simulink model "disk drive adaptive control"  (R2020a)
settings: Solver=VariableStepAuto  StartTime=0.0  StopTime=100  RelTol=1e-13  AbsTol=1e-8
InitFcn:
  | A1=2*rand(1);
  | A2=4*rand(1);
  | w1=1;w2=3;
  | phi1=2*pi*rand(1);
  | phi2=2*pi*rand(1);
  | Kp=1;
  | gamma=10;
  | A1ref=3;
  | A2ref=2;
  | w1ref=2;w2ref=sqrt(3);
  | phi1ref=0;
  | phi2ref=pi/4;
settings Model: Creator=Haris  LastModifiedBy=Haris

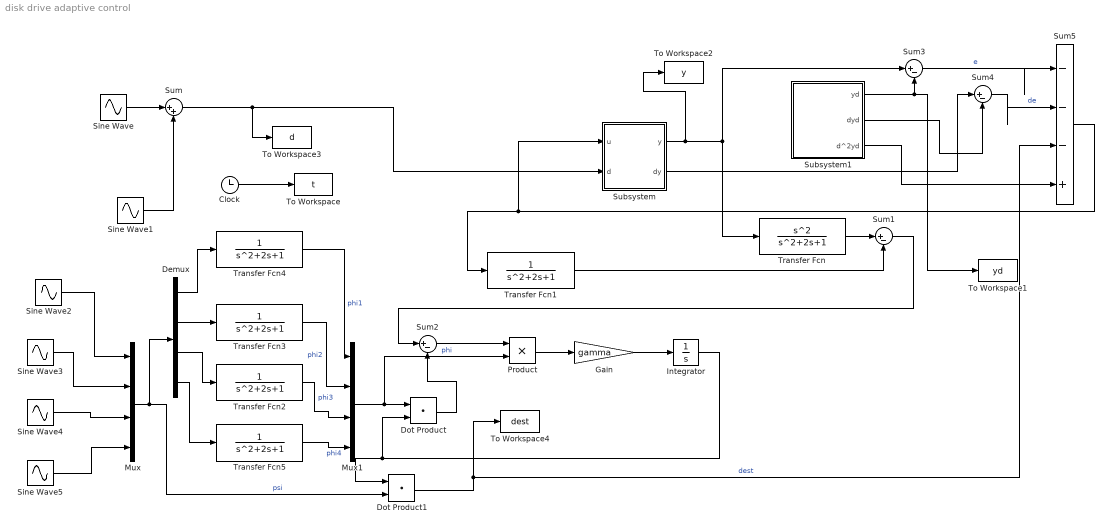
== system disk drive adaptive control ==
  Clock : Clock
  Demux : Demux
  Dot Product : DotProduct  InputSameDT=on  OutDataTypeStr=Inherit: Inherit via internal rule
  Dot Product1 : DotProduct  InputSameDT=on  OutDataTypeStr=Inherit: Inherit via internal rule
  Gain : Gain  Gain=gamma
  Integrator : Integrator  InitialCondition=[0;0;0;0]
  Mux : Mux
  Mux1 : Mux
  Product : Product
  Sine Wave : Sin  Amplitude=A1  Frequency=w1  Phase=phi1  SampleTime=0
  Sine Wave1 : Sin  Amplitude=A2  Frequency=w2  Phase=phi2  SampleTime=0
  Sine Wave2 : Sin  Frequency=w1  SampleTime=0
  Sine Wave3 : Sin  Frequency=w1  Phase=pi/2  SampleTime=0
  Sine Wave4 : Sin  Frequency=w2  SampleTime=0
  Sine Wave5 : Sin  Frequency=w2  Phase=pi/2  SampleTime=0
  Subsystem : Subsystem
  Subsystem1 : Subsystem
  Sum : Sum  Inputs=|++
  Sum{1..4} (4 alike) : Sum  Inputs=|+-
  Sum5 : Sum  Inputs=|---+
  To Workspace : ToWorkspace  VariableName=t  SampleTime=-1
  To Workspace1 : ToWorkspace  VariableName=yd  SampleTime=-1
  To Workspace2 : ToWorkspace  VariableName=y  SampleTime=-1
  To Workspace3 : ToWorkspace  VariableName=d  SampleTime=-1
  To Workspace4 : ToWorkspace  VariableName=dest  SampleTime=-1
  Transfer Fcn : TransferFcn  Numerator=[1 0 0]
  Transfer Fcn{1..5} (5 alike) : TransferFcn
  wires:
  Sine Wave/1 -> Sum/1
  Sine Wave1/1 -> Sum/2
  Sum/1 -> To Workspace3/1, Subsystem/2(d)
  Subsystem/1(y) -> To Workspace2/1, Transfer Fcn/1, Sum3/1
  Sum5/1 -> Subsystem/1(u), Transfer Fcn1/1
  Transfer Fcn/1 -> Sum1/1
  Transfer Fcn1/1 -> Sum1/2
  Sum1/1 -> Sum2/1
  Gain/1 -> Integrator/1
  Sine Wave2/1 -> Mux/1
  Sine Wave3/1 -> Mux/2
  Sine Wave4/1 -> Mux/3
  Sine Wave5/1 -> Mux/4
  Mux/1 -> Demux/1, Dot Product1/2  "psi"
  Integrator/1 -> Dot Product/2, Dot Product1/1
  Dot Product/1 -> Sum2/2
  Sum2/1 -> Product/1
  Product/1 -> Gain/1
  Dot Product1/1 -> To Workspace4/1, Sum5/3  "dest"
  Subsystem1/1(yd) -> To Workspace1/1, Sum3/2
  Subsystem1/2(dyd) -> Sum4/2
  Subsystem/2(dy) -> Sum4/1
  Subsystem1/3(d^2yd) -> Sum5/4
  Sum3/1 -> Sum5/1  "e"
  Sum4/1 -> Sum5/2  "de"
  Clock/1 -> To Workspace/1
  Mux1/1 -> Product/2, Dot Product/1  "phi"
  Demux/1 -> Transfer Fcn4/1
  Demux/2 -> Transfer Fcn3/1
  Demux/3 -> Transfer Fcn2/1
  Demux/4 -> Transfer Fcn5/1
  Transfer Fcn4/1 -> Mux1/1  "phi1"
  Transfer Fcn3/1 -> Mux1/2  "phi2"
  Transfer Fcn2/1 -> Mux1/3  "phi3"
  Transfer Fcn5/1 -> Mux1/4  "phi4"

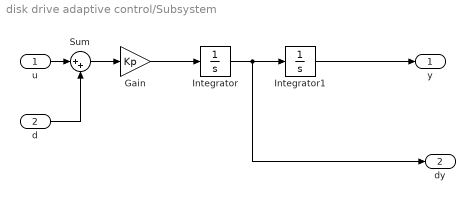
== system disk drive adaptive control/Subsystem ==
  u : Inport
  d : Inport  Port=2
  Gain : Gain  Gain=Kp
  Integrator : Integrator
  Integrator1 : Integrator
  Sum : Sum  Inputs=|++
  y : Outport
  dy : Outport  Port=2
  wires:
  Integrator1/1 -> y/1
  Gain/1 -> Integrator/1
  Sum/1 -> Gain/1
  u/1 -> Sum/1
  Integrator/1 -> dy/1, Integrator1/1
  d/1 -> Sum/2

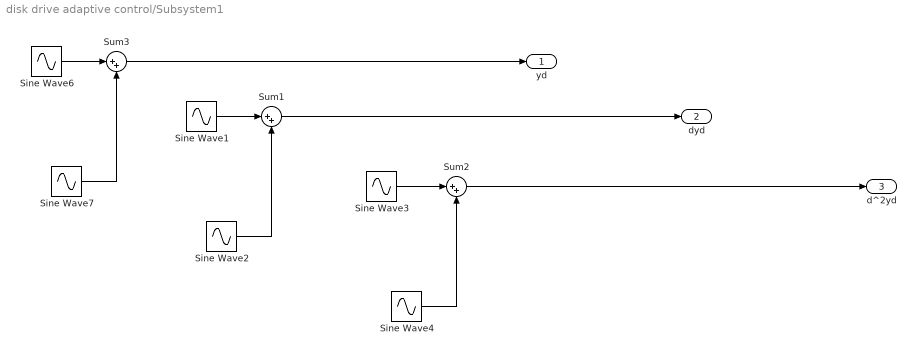
== system disk drive adaptive control/Subsystem1 ==
  Sine Wave1 : Sin  Amplitude=A1ref*w1ref  Frequency=w1ref  Phase=phi1ref+pi/2  SampleTime=0
  Sine Wave2 : Sin  Amplitude=A2ref*w2ref  Frequency=w2ref  Phase=phi2ref+pi/2  SampleTime=0
  Sine Wave3 : Sin  Amplitude=A1ref*w1ref^2  Frequency=w1ref  Phase=phi1ref+pi  SampleTime=0
  Sine Wave4 : Sin  Amplitude=A2ref*w2ref^2  Frequency=w2ref  Phase=phi2ref+pi  SampleTime=0
  Sine Wave6 : Sin  Amplitude=A1ref  Frequency=w1ref  Phase=phi1ref  SampleTime=0
  Sine Wave7 : Sin  Amplitude=A2ref  Frequency=w2ref  Phase=phi2ref  SampleTime=0
  Sum1 : Sum  Inputs=|++
  Sum2 : Sum  Inputs=|++
  Sum3 : Sum  Inputs=|++
  yd : Outport
  dyd : Outport  Port=2
  d^2yd : Outport  Port=3
  wires:
  Sine Wave7/1 -> Sum3/2
  Sum3/1 -> yd/1
  Sine Wave6/1 -> Sum3/1
  Sum1/1 -> dyd/1
  Sine Wave2/1 -> Sum1/2
  Sine Wave1/1 -> Sum1/1
  Sum2/1 -> d^2yd/1
  Sine Wave4/1 -> Sum2/2
  Sine Wave3/1 -> Sum2/1
